simulink model "HW3_model"  (R2021b)
settings: Solver=ode4  StartTime=0.0  StopTime=3  FixedStep=.005  RelTol=1e-3
values from neighbouring files (symbols this model uses):
  A = double(subs(jacobian(f,[x1;x2;x3;x4;x5;x6]),[x1;x2;x3;x4;x5;x6;u1;u2;u3],[xe;ue]))    [HW3.m]
  B = double(subs(jacobian(f,[u1;u2;u3]),[x1;x2;x3;x4;x5;x6;u1;u2;u3],[xe;ue]))    [HW3.m]
  C = double(jacobian(h,[x1;x2;x3;x4;x5;x6]))    [HW3.m]
  D = double(jacobian(h,[u1;u2;u3]))    [HW3.m]
  K = Z/S    [HW3.m]
  L = (m2*(x_dot(t) + L1*cos(theta1(t))*theta_dot_1(t) + L2*cos(theta2(t))*        theta_dot_2(t))^2)/2 + (m1*(x_dot(t) + L1*cos(theta1(t))*        theta_dot_1(t))^2)/2 + (m2*(L1*sin(theta1(t))*theta_dot_1(t) +        L2*sin(theta2(t))*theta_dot_2(t))^2)/2 + (M*x_dot(t)^2)/2 +         (L1^2*m1*sin(theta1(t))^2*theta_dot_1(t)^2)/2 -         L1*g*m1*cos(theta1(t)) - L1*g*m2*cos(theta1(t)) - L2*g*m2*cos(th ...(+8 chars)    [HW3.m]
  ue = fsolve(fun,[0 0 0]',fsol_opt)    [HW3.m]
  x0 = [0 .01 .02 0 0 0]'    [HW3.m]
  xe = [0.1, deg2rad(60), deg2rad(45),  0, 0, 0 ]'    [HW3.m]
  ye = double(subs(h,[x1;x2;x3;x4;x5;x6],xe))    [HW3.m]
libraries: vrlib x1
settings Model: Creator=17165  LastModifiedBy=17165

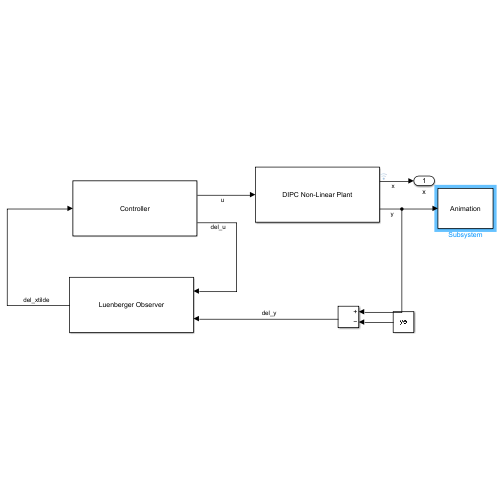
[thumbnail: Simulink's stored preview of the top-level diagram]
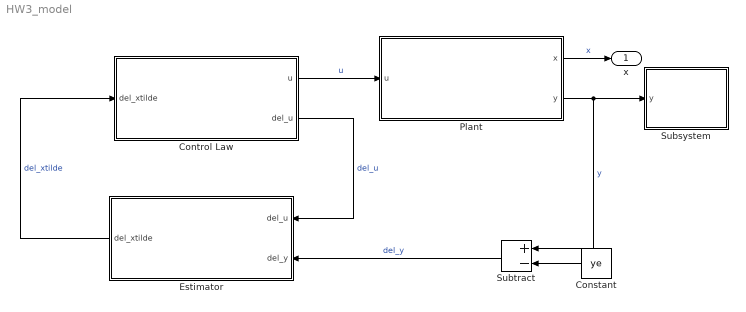
== system HW3_model ==
  Constant : Constant  Value=ye
  Control Law : Subsystem
      mask Display: disp('Controller')
  Estimator : Subsystem
      mask Display: disp('Luenberger Observer')
  Plant : Subsystem
      mask Display: disp('DIPC Non-Linear Plant')
  Subsystem : Subsystem
      mask Display: disp('Animation')
  Subtract : Sum  Inputs=+-
  x : Outport
  wires:
  Control Law/1(u) -> Plant/1(u)  "u"
  Plant/2(y) -> Subtract/1, Subsystem/1(y)  "y"
  Constant/1 -> Subtract/2
  Subtract/1 -> Estimator/2(del_y)  "del_y"
  Estimator/1(del_xtilde) -> Control Law/1(del_xtilde)  "del_xtilde"
  Control Law/2(del_u) -> Estimator/1(del_u)  "del_u"
  Plant/1(x) -> x/1  "x"

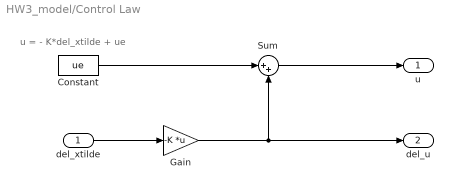
== system HW3_model/Control Law ==
  note: u = - K*del_xtilde + ue
  del_xtilde : Inport
  Constant : Constant  Value=ue
  Gain : Gain  Gain=-K  Multiplication=Matrix(K*u)
  Sum : Sum  Inputs=|++
  u : Outport
  del_u : Outport  Port=2
  wires:
  del_xtilde/1 -> Gain/1
  Gain/1 -> Sum/2, del_u/1
  Sum/1 -> u/1
  Constant/1 -> Sum/1

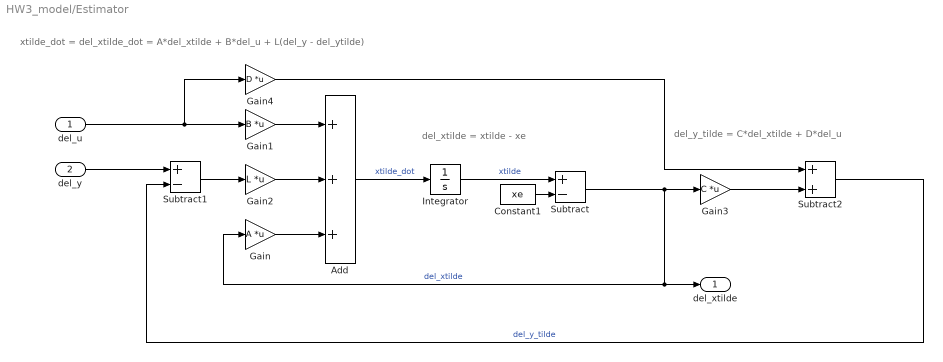
== system HW3_model/Estimator ==
  note: del_y_tilde = C*del_xtilde + D*del_u
  note: del_xtilde = xtilde - xe
  note: xtilde_dot = del_xtilde_dot = A*del_xtilde + B*del_u + L(del_y - del_ytilde)
  del_u : Inport
  del_y : Inport  Port=2
  Add : Sum  Inputs=+++
  Constant1 : Constant  Value=xe
  Gain : Gain  Gain=A  Multiplication=Matrix(K*u)
  Gain1 : Gain  Gain=B  Multiplication=Matrix(K*u)
  Gain2 : Gain  Gain=L  Multiplication=Matrix(K*u)
  Gain3 : Gain  Gain=C  Multiplication=Matrix(K*u)
  Gain4 : Gain  Gain=D  Multiplication=Matrix(K*u)
  Integrator : Integrator
  Subtract : Sum  Inputs=+-
  Subtract1 : Sum  Inputs=+-
  Subtract2 : Sum
  del_xtilde : Outport
  wires:
  Gain1/1 -> Add/1
  Add/1 -> Integrator/1  "xtilde_dot"
  Gain/1 -> Add/3
  Gain2/1 -> Add/2
  Subtract1/1 -> Gain2/1
  Gain3/1 -> Subtract2/2
  Gain4/1 -> Subtract2/1
  Subtract2/1 -> Subtract1/2  "del_y_tilde"
  del_u/1 -> Gain4/1, Gain1/1
  del_y/1 -> Subtract1/1
  Constant1/1 -> Subtract/2
  Integrator/1 -> Subtract/1  "xtilde"
  Subtract/1 -> del_xtilde/1, Gain/1, Gain3/1  "del_xtilde"

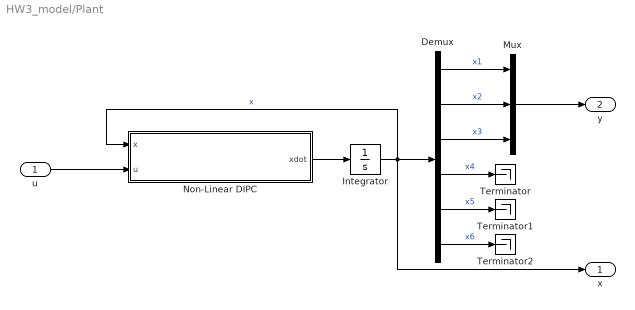
== system HW3_model/Plant ==
  u : Inport
  Demux : Demux  Outputs=6
  Integrator : Integrator  InitialCondition=x0
  Mux : Mux  Inputs=3
  Non-Linear DIPC : MATLAB Function  TreatAsAtomicUnit=on
  Terminator : Terminator
  Terminator1 : Terminator
  Terminator2 : Terminator
  x : Outport
  y : Outport  Port=2
  wires:
  Demux/6 -> Terminator2/1  "x6"
  u/1 -> Non-Linear DIPC/2(u)
  Mux/1 -> y/1
  Demux/5 -> Terminator1/1  "x5"
  Non-Linear DIPC/1(xdot) -> Integrator/1
  Demux/1 -> Mux/1  "x1"
  Integrator/1 -> x/1, Non-Linear DIPC/1(x), Demux/1  "x"
  Demux/4 -> Terminator/1  "x4"
  Demux/3 -> Mux/3  "x3"
  Demux/2 -> Mux/2  "x2"

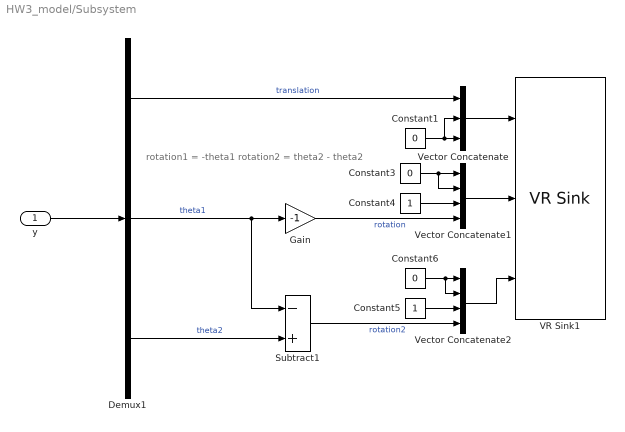
== system HW3_model/Subsystem ==
  note: rotation1 = -theta1
      | rotation2 = theta2 - theta2
  y : Inport
  Constant1 : Constant  Value=0
  Constant3 : Constant  Value=0
  Constant4 : Constant
  Constant5 : Constant
  Constant6 : Constant  Value=0
  Demux1 : Demux  Outputs=3
  Gain : Gain  Gain=-1
  Subtract1 : Sum  Inputs=-+
  VR Sink1 : vrlib/VR Sink  InstantiateOnLoad=on  SampleTime=.005  ViewEnable=on  RemoteChange=off  RemoteView=off  FieldsWritten=Cart.translation.3.1.1.double#Rotation1.rotation.4.1.1.double#Rotation2.rotation.4.1.1.double  WorldFileName=DIPC.x3d  AutoView=off  VideoDimensions=[]  AllowVariableSize=off
  Vector Concatenate : Concatenate  NumInputs=3
  Vector Concatenate1 : Concatenate  NumInputs=4
  Vector Concatenate2 : Concatenate  NumInputs=4
  wires:
  Constant3/1 -> Vector Concatenate1/2, Vector Concatenate1/1
  Gain/1 -> Vector Concatenate1/4  "rotation"
  Constant4/1 -> Vector Concatenate1/3
  Constant1/1 -> Vector Concatenate/2, Vector Concatenate/3
  Demux1/2 -> Subtract1/1, Gain/1  "theta1"
  Demux1/3 -> Subtract1/2  "theta2"
  y/1 -> Demux1/1
  Subtract1/1 -> Vector Concatenate2/4  "rotation2"
  Vector Concatenate1/1 -> VR Sink1/2
  Vector Concatenate2/1 -> VR Sink1/3
  Vector Concatenate/1 -> VR Sink1/1
  Demux1/1 -> Vector Concatenate/1  "translation"
  Constant5/1 -> Vector Concatenate2/3
  Constant6/1 -> Vector Concatenate2/2, Vector Concatenate2/1

== matlab function HW3_model/Plant/Non-Linear DIPC ==
  data: x input; u input; xdot output
function xdot = DIPC_Simulink(x, u)
% Define State and Input Vectors
x1          = x(1,1);  % x
x2          = x(2,1);  % theta_1
x3          = x(3,1);  % theta_2
x4          = x(4,1);  % xdot
x5          = x(5,1);  % theta_1_dot
x6          = x(6,1);  % theta_2_dot
u1          = u(1,1);
u2          = u(2,1);
u3          = u(3,1);

m1  = 0.5;
L1  = 0.5;
m2  = 0.75;
L2  = 0.75;
M   = 1.5;
g   = 9.81;


% State Dynamics
x1dot       = x4;   % xdot
x2dot       = x5;   % theta_1_dot
x3dot       = x6;   % theta_2_dot

% x_ddot
x4dot       = (L2*m2*u2*cos(x2 - 2*x3) - L1*m1*u3*cos(x3) - L2*m2*u2*cos(x2)...
               - L1*m2*u3*cos(x3) - 2*L2*m1*u2*cos(x2) + 2*L1*L2*m1*u1 + L1*L2*m2*u1...
               + L1*m1*u3*cos(2*x2 - x3) + L1*m2*u3*cos(2*x2 - x3) -...
               L1*L2*m2*u1*cos(2*x2 - 2*x3) - L1*L2*g*m1^2*sin(2*x2) +...
               2*L1^2*L2*m1^2*x5^2*sin(x2) - L1*L2*g*m1*m2*sin(2*x2) +...
               L1*L2^2*m1*m2*x6^2*sin(2*x2 - x3) + 2*L1^2*L2*m1*m2*x5^2*sin(x2) +...
               L1*L2^2*m1*m2*x6^2*sin(x3))/(L1*L2*(2*M*m1 + M*m2 + m1*m2 -...
               m1^2*cos(2*x2) + m1^2 - m1*m2*cos(2*x2) - M*m2*cos(2*x2 - 2*x3)));
 
% theta_1_ddot
x5dot       = -(L2*m2*u2*cos(2*x3) - 2*L2*m1*u2 - L2*m2*u2 - 2*L2*M*u2 -...
                2*L1*L2*g*m1^2*sin(x2) + 2*L1*M*u3*cos(x2)*cos(x3) +...
                2*L1*M*u3*sin(x2)*sin(x3) + L1^2*L2*m1^2*x5^2*sin(2*x2) +...
                2*L1*m1*u3*sin(x2)*sin(x3) + 2*L1*m2*u3*sin(x2)*sin(x3) +...
                2*L1*L2*m1*u1*cos(x2) + L1*L2*m2*u1*cos(x2) - 2*L1*L2*M*g*m1*sin(x2)...
                - L1*L2*M*g*m2*sin(x2) - L1*L2*m2*u1*sin(2*x3)*sin(x2) -...
                2*L1*L2*g*m1*m2*sin(x2) + L1^2*L2*m1*m2*x5^2*sin(2*x2) -...
                L1*L2*m2*u1*cos(2*x3)*cos(x2) - L1*L2*M*g*m2*cos(2*x3)*sin(x2) +...
                L1*L2*M*g*m2*sin(2*x3)*cos(x2) - L1^2*L2*M*m2*x5^2*cos(2*x2)*sin(2*x3) +...
                L1^2*L2*M*m2*x5^2*cos(2*x3)*sin(2*x2) - 2*L1*L2^2*M*m2*x6^2*cos(x2)*sin(x3) +...
                2*L1*L2^2*M*m2*x6^2*cos(x3)*sin(x2) + 2*L1*L2^2*m1*m2*x6^2*cos(x3)*sin(x2))/...
                (L1^2*L2*(2*M*m1 + M*m2 + m1*m2 - m1^2*cos(2*x2) + m1^2 -...
                m1*m2*cos(2*x2) - M*m2*cos(2*x2 - 2*x3)));


% theta_2_ddot
x6dot       = (L1*m1^2*u3 + L1*m2^2*u3 - L1*m1^2*u3*cos(2*x2) - L1*m2^2*u3*cos(2*x2) +...
              L2*m2^2*u2*cos(x2 + x3) + 2*L1*M*m1*u3 + 2*L1*M*m2*u3 + 2*L1*m1*m2*u3 -...
              L2*m2^2*u2*cos(x2 - x3) - L2*m1*m2*u2*cos(x2 - x3) - L1*L2*m2^2*u1*cos(x3) -...
              2*L1*m1*m2*u3*cos(2*x2) + L1*L2*m2^2*u1*cos(2*x2 - x3) +...
              L2*m1*m2*u2*cos(x2 + x3) - 2*L2*M*m2*u2*cos(x2 - x3) - L1*L2*m1*m2*u1*cos(x3) +...
              L1*L2*M*g*m2^2*sin(x3) + 2*L1^2*L2*M*m2^2*x5^2*sin(x2 - x3) +...
              L1*L2*m1*m2*u1*cos(2*x2 - x3) + L1*L2^2*M*m2^2*x6^2*sin(2*x2 - 2*x3) -...
              L1*L2*M*g*m2^2*sin(2*x2 - x3) - L1*L2*M*g*m1*m2*sin(2*x2 - x3) +...
              L1*L2*M*g*m1*m2*sin(x3) + 2*L1^2*L2*M*m1*m2*x5^2*sin(x2 - x3))/...
              (L1*L2^2*m2*(2*M*m1 + M*m2 + m1*m2 - m1^2*cos(2*x2) + m1^2 -...
              m1*m2*cos(2*x2) - M*m2*cos(2*x2 - 2*x3)));


xdot        = [x1dot;x2dot;x3dot;x4dot;x5dot;x6dot];

end
